simulink library "FilterLib"  (R2022a)
settings: Solver=VariableStepAuto  StartTime=0.0  StopTime=10.0  RelTol=1e-3
Description:
  | This block library contains common filters for use by models in the project.
settings Model: Creator=The MathWorks, Inc.  LastModifiedBy=manthony
settings SolverCC: AlgebraicLoopSolver=TrustRegion
settings DataIOCC: ReturnWorkspaceOutputs=off
settings DebuggingCC: UnconnectedInputMsg=warning  UnconnectedOutputMsg=warning  UnconnectedLineMsg=warning  PregeneratedLibrarySubsystemCodeDiagnostic=none  SFMachineParentedDataDiag=warning  ArithmeticOperatorsInVariantConditions=warning
settings SFSimCC: SimUseLocalCustomCode=off  CustomCodeUndefinedFunction=UseInterfaceOnly
settings RTWCC: RTWUseLocalCustomCode=off  DLArmComputeVersion=19.05
settings CodeAppCC: StateflowObjectComments=on

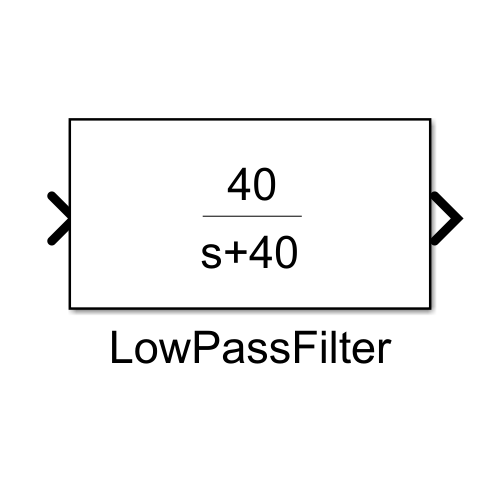
[thumbnail: Simulink's stored preview of the top-level diagram]
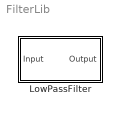
== system FilterLib ==
  LowPassFilter : Subsystem  Tag=FilterWizardSubSystem  mask(Low Pass Filter){fq=40, ts=0.01}
      mask prompts: fq "Roll-off frequency (rad/s)"; ts "Sample time"
      mask help: Discrete low pass filter.
      mask init:
      | n2 = 1;
      | d2 = 1;
      | num = fq;
      | den = [1,fq];
      | contSys = tf(num,den);
      | if ts > 0
      |     discSys = c2d(contSys,ts);
      |     [n,d] = tfdata(discSys,'v');
      |     n2 = n(2);
      |     d2 = -d(2);
      | else
      |     error('Please specify a discrete sample time.');
      | end
      settings: ErrorFcn=dspFilterRealizedInBasicElemsAlgLoopErrFcnCallback
      mask Display: dpoly([0,fq],[1,fq]);

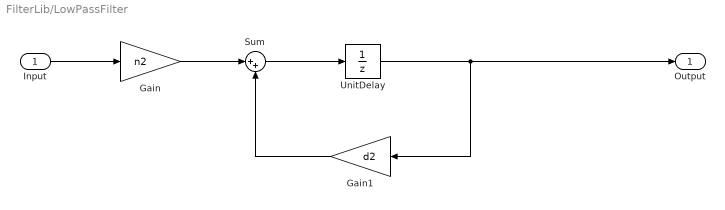
== system FilterLib/LowPassFilter ==
  Input : Inport
  Gain : Gain  Gain=n2
  Gain1 : Gain  Gain=d2
  Sum : Sum  Inputs=|++
  UnitDelay : UnitDelay  SampleTime=ts  HasFrameUpgradeWarning=on
  Output : Outport  VectorParamsAs1DForOutWhenUnconnected=off
  wires:
  Input/1 -> Gain/1
  Gain1/1 -> Sum/2
  Sum/1 -> UnitDelay/1
  Gain/1 -> Sum/1
  UnitDelay/1 -> Output/1, Gain1/1
